simulink model "EPT"  (R2019b)
settings: Solver=FixedStepDiscrete  StartTime=0.0  StopTime=5  FixedStep=0.005  RelTol=1e-3  EnableMultiTasking=on
PreLoadFcn:
  | try, model_open; catch, disp('Error occurred while executing model pre-load callback: model_open.m'); disp('Please assure that the MATLAB working directory is set to the model directory before opening.'); end
InitFcn:
  | try, model_open; catch, end
undefined symbols (not defined in the file or in its folder): Bridge, GCM, H, ln, raptor_get_param_eval, raptor_get_safe_string, raptor_xcp_function
libraries: Raptor_lib x2810, simulink x374, hdlsllib x19
(part 20 of 45)

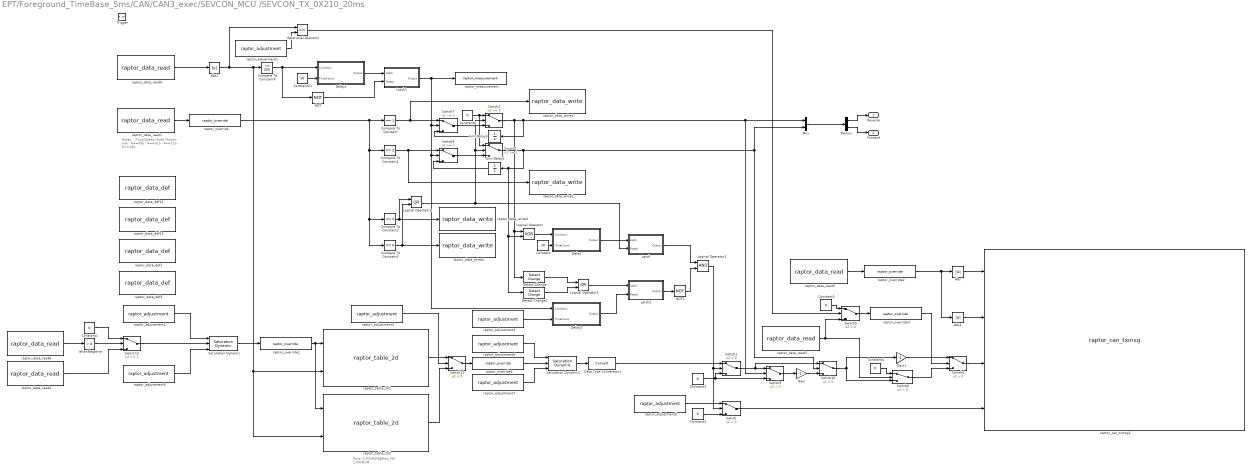
== system EPT/Foreground_TimeBase_5ms/CAN/CAN3_exec/SEVCON_MCU /SEVCON_TX_0X210_20ms  ==
  note: Note:
      | 0:FOXNUM@New_FW
      | 1:FOXNUM
  note: Notes :
      | - Torq/Speed Mode Chosen one
      | - N==00b
      | - R==01b
      | - P==11b
      | - D==10b
  Trigger : TriggerPort  VariantControl=Variant  PortDimensions=1
  Abs : Abs
  Abs1 : Abs
  Abs2 : Abs
  Compare To Constant : simulink/Logic and Bit Operations/Compare To Constant  relop===  const=1  OutDataTypeStr=boolean
  Compare To Constant1 : simulink/Logic and Bit Operations/Compare To Constant  relop===  const=2  OutDataTypeStr=boolean
  Compare To Constant2 : simulink/Logic and Bit Operations/Compare To Constant  relop===  const=3  OutDataTypeStr=boolean
  Compare To Constant3 : simulink/Logic and Bit Operations/Compare To Constant  relop===  const=0  OutDataTypeStr=boolean
  Compare To Constant4 : simulink/Logic and Bit Operations/Compare To Constant  relop=<=  const=200  OutDataTypeStr=boolean
  Constant : Constant  Value=10
  Constant{1..5} (5 alike) : Constant  Value=0
  Constant21 : Constant  Value=10
  Constant6 : Constant  Value=0  OutDataTypeStr=boolean
  Data Type Conversion1 : DataTypeConversion
  Delay : Subsystem
  Delay1 : Subsystem
  Delay3 : Subsystem
  Demux : Demux  Outputs=2
  Detect Change : simulink/Logic and Bit Operations/Detect Change  vinit=0  OutDataTypeStr=boolean
  Detect Change1 : simulink/Logic and Bit Operations/Detect Change  vinit=0  OutDataTypeStr=boolean
  Gain : Gain  Gain=-1
  Gain1 : Gain  Gain=-1
  IsNonNegative : simulink/Logic and Bit Operations/Compare To Zero  relop=>  OutDataTypeStr=boolean
  Latch : Subsystem
  Latch1 : Subsystem
  Latch2 : Subsystem
  Logical Operator : Logic  Operator=XOR  AllPortsSameDT=off  OutDataTypeStr=boolean
  Logical Operator1 : Logic  Operator=OR  AllPortsSameDT=off  OutDataTypeStr=boolean
  Logical Operator2 : Logic  Operator=OR  AllPortsSameDT=off  OutDataTypeStr=boolean
  Logical Operator3 : Logic  AllPortsSameDT=off  OutDataTypeStr=boolean
  Mux : Mux  Inputs=2
  NOT : Logic  Operator=NOT  IconShape=distinctive  AllPortsSameDT=off  OutDataTypeStr=boolean
  NOT1 : Logic  Operator=NOT  IconShape=distinctive  AllPortsSameDT=off  OutDataTypeStr=boolean
  Relational Operator : RelationalOperator  Operator=<=  OutDataTypeStr=boolean  RndMeth=Simplest
  Saturation Dynamic : simulink/Discontinuities/Saturation Dynamic  OutMin=[]  OutMax=[]  OutDataTypeStr=Inherit: Same as second input  OutDataType=fixdt(1, 16)  OutScaling=2^-10  DoSatur=off
  Saturation Dynamic1 : simulink/Discontinuities/Saturation Dynamic  OutMin=[]  OutMax=[]  OutDataTypeStr=Inherit: Same as second input  OutDataType=fixdt(1, 16)  OutScaling=2^-10  DoSatur=off
  Switch{,1,4..6,9..11} (8 alike) : Switch  Criteria=u2 > Threshold
  Switch{2..3,7..8,12} (5 alike) : Switch  Threshold=1
  Unit Delay1 : UnitDelay  SampleTime=-1  HasFrameUpgradeWarning=on
  Unit Delay3 : UnitDelay  SampleTime=-1  HasFrameUpgradeWarning=on
  raptor_adjustment1 : Raptor_lib/Data Storage/raptor_adjustment  paramName='Cal_Regen_Speed'  nameSource=Parameter  initValue=1000  dataType=double  storage=Calibration  calDispType=Number  calEnum={'False', 'True'}  calGain=1.0  calOffset=0.0  calMax=inf  calMin=-inf  calFormat='-1'  calUnit=''  calHelp=''  calAccess=1  calFunction=raptor_xcp_function(gcb)  calDispHeaders=off  calColHeaders={'Col1' 'Col2' 'Col3'}  calRowHeaders={'Row1' 'Row2' 'Row3'}
      settings: SourceProductName=Raptor
  raptor_adjustment2 : Raptor_lib/Data Storage/raptor_adjustment  paramName='Cal_TorqueMax'  nameSource=Parameter  initValue=150  dataType=double  storage=Calibration  calDispType=Number  calEnum={'False', 'True'}  calGain=1.0  calOffset=0.0  calMax=150  calMin=-150  calFormat='-1'  calUnit=''  calHelp=''  calAccess=1  calFunction=raptor_xcp_function(gcb)  calDispHeaders=off  calColHeaders={'Col1' 'Col2' 'Col3'}  calRowHeaders={'Row1' 'Row2' 'Row3'}
      settings: SourceProductName=Raptor
  raptor_adjustment3 : Raptor_lib/Data Storage/raptor_adjustment  paramName='Cal_Motor_Select'  nameSource=Parameter  initValue=1  dataType=boolean  storage=Calibration  calDispType=Number  calEnum={'False', 'True'}  calGain=1.0  calOffset=0.0  calMax=inf  calMin=-inf  calFormat='-1'  calUnit=''  calHelp=''  calAccess=1  calFunction=raptor_xcp_function(gcb)  calDispHeaders=off  calColHeaders={'Col1' 'Col2' 'Col3'}  calRowHeaders={'Row1' 'Row2' 'Row3'}
      settings: SourceProductName=Raptor
  raptor_adjustment4 : Raptor_lib/Data Storage/raptor_adjustment  paramName='Cal_Torque_Output_DelayTimes'  nameSource=Parameter  initValue=10  dataType=double  storage=Calibration  calDispType=Number  calEnum={'False', 'True'}  calGain=1.0  calOffset=0.0  calMax=inf  calMin=-inf  calFormat='-1'  calUnit=''  calHelp=''  calAccess=1  calFunction=raptor_xcp_function(gcb)  calDispHeaders=off  calColHeaders={'Col1' 'Col2' 'Col3'}  calRowHeaders={'Row1' 'Row2' 'Row3'}
      settings: SourceProductName=Raptor
  raptor_adjustment5 : Raptor_lib/Data Storage/raptor_adjustment  paramName='Cmd_Throttle_Inlet_voltage'  nameSource=Parameter  initValue=3  dataType=double  storage=Calibration  calDispType=Number  calEnum={'False', 'True'}  calGain=1.0  calOffset=0.0  calMax=inf  calMin=0  calFormat='-1'  calUnit=''  calHelp=''  calAccess=1  calFunction=raptor_xcp_function(gcb)  calDispHeaders=off  calColHeaders={'Col1' 'Col2' 'Col3'}  calRowHeaders={'Row1' 'Row2' 'Row3'}
      settings: SourceProductName=Raptor
  raptor_adjustment6 : Raptor_lib/Data Storage/raptor_adjustment  paramName='Cal_Cmd_Torque_Percentage_Max'  nameSource=Parameter  initValue=100  dataType=double  storage=Calibration  calDispType=Number  calEnum={'False', 'True'}  calGain=1.0  calOffset=0.0  calMax=inf  calMin=-inf  calFormat='-1'  calUnit=''  calHelp=''  calAccess=1  calFunction=raptor_xcp_function(gcb)  calDispHeaders=off  calColHeaders={'Col1' 'Col2' 'Col3'}  calRowHeaders={'Row1' 'Row2' 'Row3'}
      settings: SourceProductName=Raptor
  raptor_adjustment7 : Raptor_lib/Data Storage/raptor_adjustment  paramName='Cal_Cmd_Torque_Percentage_Min'  nameSource=Parameter  initValue=0  dataType=double  storage=Calibration  calDispType=Number  calEnum={'False', 'True'}  calGain=1.0  calOffset=0.0  calMax=inf  calMin=-inf  calFormat='-1'  calUnit=''  calHelp=''  calAccess=1  calFunction=raptor_xcp_function(gcb)  calDispHeaders=off  calColHeaders={'Col1' 'Col2' 'Col3'}  calRowHeaders={'Row1' 'Row2' 'Row3'}
      settings: SourceProductName=Raptor
  raptor_adjustment9 : Raptor_lib/Data Storage/raptor_adjustment  paramName='Cal_TorqueMin'  nameSource=Parameter  initValue=0.00  dataType=double  storage=Calibration  calDispType=Number  calEnum={'False', 'True'}  calGain=1.0  calOffset=0.0  calMax=150  calMin=-150  calFormat='-1'  calUnit=''  calHelp=''  calAccess=1  calFunction=raptor_xcp_function(gcb)  calDispHeaders=off  calColHeaders={'Col1' 'Col2' 'Col3'}  calRowHeaders={'Row1' 'Row2' 'Row3'}
      settings: SourceProductName=Raptor
  raptor_can_txmsg1 : Raptor_lib/CAN/raptor_can_txmsg  canDefinition=struct('dbcFile', 'SEVCON_Controller_CANopen.dbc','message', 'Cmd2','comment', '','signals', {{'Cmd_Maximum_Speed_in_Reverse','Cmd_Maximum_Speed_in_Forward','Cmd_Target_Torque','Cmd_Throttle_Inlet_voltage'}},'enabled', [ 1 1 1 1;],'canBus', '''CAN3''','messageID', [ 528;],'idMask', [ 536870911;],'payloadMask', [],'payloadValue', [],'period', [ 0;],'mailbox', '','queueSize', [ 1;],'label', [ 0;],'ver', [ 2;],'showID', [ 0;],'showRaw', [ 0;],'fill', [ 0;],'editID', [ 0;],'signalOrder', [ 2;])  canBus='CAN3'  queueSize=1  payloadMask=[]  payloadValue=[]  period=0  showID=0  label=0  idMask=hex2dec('1FFFFFFF')  fill=0  id=528  showRaw=0  signalOrder=2  signalInfo={{struct('Name', 'Cmd_Throttle_Inlet_voltage','Startbit', [ 0;],'SignalSize', [ 16;],'ByteOrder', 'LittleEndian','ValueType', 'SIGNED','Class', 'int16','Signed', [ 1;],'Factor', [ 0.0039;],'Offset', [ 0;],'Min', [ 0;],'Max', [ 0;],'Units', '','Comment', '','StartBit', [ 0;]),struct('Name', 'Cmd_Target_Torque','Startbit', [ 0;],'SignalSize', [ 16;],'ByteOrder', 'LittleEndian','ValueType', 'SIGNED','Class', 'int16','Signed', [ 1;],'Factor', [ 0.1;],'Offset', [ 0;],'Min', [ 0;],'Max', [ 0;],'Units', '','Comment', '','StartBit', [ 16;]),struct('Name', 'Cmd_Maximum_Speed_in_Reverse','Startbit', [ 0;],'SignalSize', [ 16;],'ByteOrder', 'LittleEndian','ValueType', 'SIGNED','Class', 'int16','Signed', [ 1;],'Factor', [ 1;],'Offset', [ 0;],'Min', [ 0;],'Max', [ 0;],'Units', '','Comment', '','StartBit', [ 48;]),struct('Name', 'Cmd_Maximum_Speed_in_Forward','Startbit', [ 0;],'SignalSize', [ 16;],'ByteOrder', 'LittleEndian','ValueType', 'SIGNED','Class', 'int16','Signed', [ 1;],'Factor', [ 1;],'Offset', [ 0;],'Min', [ 0;],'Max', [ 0;],'Units', '','Comment', '','StartBit', [ 32;])}}
      settings: SourceProductName=Raptor
  raptor_data_def1 : Raptor_lib/Data Storage/raptor_data_def  dataName='Position_N'  initValue=0  dataType=boolean  storage=Calibration  calVisible=on  calType=Measurement  calDispType=Number  calEnum={'False', 'True'}  calGain=1.0  calOffset=0  calMin=-inf  calMax=inf  calFormat='-1'  calUnit=''  calHelp=''  calAccess=1  calFunction=raptor_xcp_function(gcb)  calDispHeaders=off  calColHeaders={'Col1' 'Col2' 'Col3'}  calRowHeaders={'Row1' 'Row2' 'Row3'}
      settings: SourceProductName=Raptor
  raptor_data_def13 : Raptor_lib/Data Storage/raptor_data_def  dataName='Position_R'  initValue=0  dataType=boolean  storage=Calibration  calVisible=on  calType=Measurement  calDispType=Number  calEnum={'False', 'True'}  calGain=1.0  calOffset=0  calMin=-inf  calMax=inf  calFormat='-1'  calUnit=''  calHelp=''  calAccess=1  calFunction=raptor_xcp_function(gcb)  calDispHeaders=off  calColHeaders={'Col1' 'Col2' 'Col3'}  calRowHeaders={'Row1' 'Row2' 'Row3'}
      settings: SourceProductName=Raptor
  raptor_data_def14 : Raptor_lib/Data Storage/raptor_data_def  dataName='Position_D'  initValue=0  dataType=boolean  storage=Calibration  calVisible=on  calType=Measurement  calDispType=Number  calEnum={'False', 'True'}  calGain=1.0  calOffset=0  calMin=-inf  calMax=inf  calFormat='-1'  calUnit=''  calHelp=''  calAccess=1  calFunction=raptor_xcp_function(gcb)  calDispHeaders=off  calColHeaders={'Col1' 'Col2' 'Col3'}  calRowHeaders={'Row1' 'Row2' 'Row3'}
      settings: SourceProductName=Raptor
  raptor_data_def3 : Raptor_lib/Data Storage/raptor_data_def  dataName='Position_P'  initValue=0  dataType=boolean  storage=Calibration  calVisible=on  calType=Measurement  calDispType=Number  calEnum={'False', 'True'}  calGain=1.0  calOffset=0  calMin=-inf  calMax=inf  calFormat='-1'  calUnit=''  calHelp=''  calAccess=1  calFunction=raptor_xcp_function(gcb)  calDispHeaders=off  calColHeaders={'Col1' 'Col2' 'Col3'}  calRowHeaders={'Row1' 'Row2' 'Row3'}
      settings: SourceProductName=Raptor
  raptor_data_read1 : Raptor_lib/Data Storage/raptor_data_read  dataName='ECHS_GEAR_CMD'  dataShape=Scalar  idxSource=Input  idxRow=1  idxCol=1
      settings: SourceProductName=Raptor
  raptor_data_read2 : Raptor_lib/Data Storage/raptor_data_read  dataName='ECHS_TRQ_CMD'  dataShape=Scalar  idxSource=Input  idxRow=1  idxCol=1
      settings: SourceProductName=Raptor
  raptor_data_read3 : Raptor_lib/Data Storage/raptor_data_read  dataName='ECHS_REG_MODE_REQ'  dataShape=Scalar  idxSource=Input  idxRow=1  idxCol=1
      settings: SourceProductName=Raptor
  raptor_data_read4 : Raptor_lib/Data Storage/raptor_data_read  dataName='Read_Motor_Speed'  dataShape=Scalar  idxSource=Input  idxRow=1  idxCol=1
      settings: SourceProductName=Raptor
  raptor_data_read5 : Raptor_lib/Data Storage/raptor_data_read  dataName='ECHS_SPD_CMD'  dataShape=Scalar  idxSource=Input  idxRow=1  idxCol=1
      settings: SourceProductName=Raptor
  raptor_data_read6 : Raptor_lib/Data Storage/raptor_data_read  dataName='HV_Off_State'  dataShape=Scalar  idxSource=Input  idxRow=1  idxCol=1
      settings: SourceProductName=Raptor
  raptor_data_write1 : Raptor_lib/Data Storage/raptor_data_write  dataName='Position_D'  dataShape=Scalar  idxSource=Input Port  idxRow=1  idxCol=1
      settings: SourceProductName=Raptor
  raptor_data_write2 : Raptor_lib/Data Storage/raptor_data_write  dataName='Position_R'  dataShape=Scalar  idxSource=Input Port  idxRow=1  idxCol=1
      settings: SourceProductName=Raptor
  raptor_data_write3 : Raptor_lib/Data Storage/raptor_data_write  dataName='Position_P'  dataShape=Scalar  idxSource=Input Port  idxRow=1  idxCol=1
      settings: SourceProductName=Raptor
  raptor_data_write4 : Raptor_lib/Data Storage/raptor_data_write  dataName='Position_N'  dataShape=Scalar  idxSource=Input Port  idxRow=1  idxCol=1
      settings: SourceProductName=Raptor
  raptor_measurement : Raptor_lib/Data Storage/raptor_measurement  paramName='FlagSpeedLow'  nameSource=Parameter  calDispType=Number  calEnum={'False', 'True'}  calGain=1.0  calOffset=0.0  calMax=inf  calMin=-inf  calFormat='-1'  calUnit=''  calHelp=''  calAccess=1  calFunction=raptor_xcp_function(gcb)  calVisible=on
      settings: SourceProductName=Raptor
  raptor_override : Raptor_lib/Data Storage/raptor_override  paramName='Cal_Cmd_F_R_Switch'  nameSource=Parameter  measurement=None  calDispType=Number  calEnum={'False', 'True'}  calGain=1.0  calOffset=0.0  calMax=inf  calMin=-inf  calFormat='-1'  calUnit=''  calHelp=''  calAccess=1  calFunction=[raptor_xcp_function(gcb) '|' raptor_get_param_eval(gcb, 'paramName') '_Override']
      settings: SourceProductName=Raptor
  raptor_override1 : Raptor_lib/Data Storage/raptor_override  paramName='Cal_Cmd_Target_Torque'  nameSource=Parameter  measurement=None  calDispType=Number  calEnum={'False', 'True'}  calGain=1.0  calOffset=0.0  calMax=inf  calMin=-inf  calFormat='-1'  calUnit=''  calHelp=''  calAccess=1  calFunction=[raptor_xcp_function(gcb) '|' raptor_get_param_eval(gcb, 'paramName') '_Override']
      settings: SourceProductName=Raptor
  raptor_override2 : Raptor_lib/Data Storage/raptor_override  paramName='Cal_Cmd_SpeedLimit'  nameSource=Parameter  measurement=None  calDispType=Number  calEnum={'False', 'True'}  calGain=1.0  calOffset=0.0  calMax=inf  calMin=-inf  calFormat='-1'  calUnit=''  calHelp=''  calAccess=1  calFunction=[raptor_xcp_function(gcb) '|' raptor_get_param_eval(gcb, 'paramName') '_Override']
      settings: SourceProductName=Raptor
  raptor_override3 : Raptor_lib/Data Storage/raptor_override  paramName='Cal_Cmd_Regen'  nameSource=Parameter  measurement=None  calDispType=Number  calEnum={'False', 'True'}  calGain=1.0  calOffset=0.0  calMax=inf  calMin=-inf  calFormat='-1'  calUnit=''  calHelp=''  calAccess=1  calFunction=[raptor_xcp_function(gcb) '|' raptor_get_param_eval(gcb, 'paramName') '_Override']
      settings: SourceProductName=Raptor
  raptor_override4 : Raptor_lib/Data Storage/raptor_override  paramName='Cal_Cmd_Torque_Percentage'  nameSource=Parameter  measurement=None  calDispType=Number  calEnum={'False', 'True'}  calGain=1.0  calOffset=0.0  calMax=inf  calMin=-inf  calFormat='-1'  calUnit=''  calHelp=''  calAccess=1  calFunction=[raptor_xcp_function(gcb) '|' raptor_get_param_eval(gcb, 'paramName') '_Override']
      settings: SourceProductName=Raptor
  raptor_table_2d1 : Raptor_lib/Table Lookup/raptor_table_2d  dataName='FOXNUM'  initValue=|  dataType=double  storage=Calibration  initValueX="[0\t500\t1000\t1500\t2000\t2500\t3000\t3500\t4000\t4500\t5000\t6000]"  initValueY="[0\t5\t10\t20\t30\t40\t50\t60\t70\t80\t90\t100\t110\t120\t130]"  dataTypeXY=double  storageXY=Calibration  calVisible=on  showTable=off  calGain=1.0  calOffset=0.0  calMax=Inf  calMin=-Inf  calFormat='-1'  calUnit=''  calHelp=''  showBreakpointX=off  dataNameX=[]  calGainX=1.0  calOffsetX=0.0  calMaxX=Inf  calMinX=-Inf  calFormatX='-1'  calUnitX=''  calHelpX=''  showBreakpointY=off  dataNameY=[]  calGainY=1.0  calOffsetY=0.0  calMaxY=Inf  calMinY=-Inf  calFormatY='-1'  calUnitY=''  calHelpY=''  calAccess=1  calFunction=raptor_xcp_function(gcb)  measureEnable=off  mName=[raptor_get_param_eval(gcb,'dataName'), '_Output']
      | [0	0	0	0	0	0	0	0	0	0	0	0
      | 26	26	26	23	21	17.5000000000000	21	19.1000000000000	17.7000000000000	17.3000000000000	16	16
      | 34	34	35	33.1000000000000	30	30	28.3000000000000	26.4000000000000	26	25	24	24
      | 44.4000000000000	44.4000000000000	46	43	39	38.3000000000000	37	35.3000000000000	34	32.5000000000000	38.5000000000000	38.5000000000000
      | 51.2000000000000	51.2000000000000	53.7000000000000	50	46	44.5000000000000	42.7000000000000	41.1000000000000	46.5000000000000	54.5000000000000	70	70
      | 59	59	60.4000000000000	56	51	50.2000000000000	48	53.9000000000000	70	100	100	100
      | 64.8000000000000	64.8000000000000	66	61	55	55	54.6000000000000	80	100	100	100	100
      | 70.3000000000000	70.3000000000000	71	65.5000000000000	58.9000000000000	59	75	100	100	100	100	100
      | 75.3000000000000	75.3000000000000	75.4000000000000	70	62.6000000000000	64.5000000000000	100	100	100	100	100	100
      | 80	80	79.9000000000000	74	68.6000000000000	85	100	100	100	100	100	100
      | 84.8000000000000	84.8000000000000	84.2000000000000	78	71.7000000000000	100	100	100	100	100	100	100
      | 89.1000000000000	89.1000000000000	88.4000000000000	81.5000000000000	81.2000000000000	100	100	100	100	100	100	100
      | 96.1000000000000	96.1000000000000	95	84	100	100	100	100	100	100	100	100
      | 100	100	100	90	100	100	100	100	100	100	100	100
      | 100	100	100	100	100	100	100	100	100	100	100	100]
      settings: SourceProductName=Raptor
  raptor_table_2d2 : Raptor_lib/Table Lookup/raptor_table_2d  dataName='AC_35'  initValue=|  dataType=double  storage=Calibration  initValueX="[0\t500\t1000\t1500\t2000\t2500\t3000\t3500\t4000\t4500\t5000\t5500\t6000\t6500]"  initValueY=|  dataTypeXY=double  storageXY=Calibration  calVisible=on  showTable=off  calGain=1.0  calOffset=0.0  calMax=Inf  calMin=-Inf  calFormat='-1'  calUnit=''  calHelp=''  showBreakpointX=off  dataNameX=[]  calGainX=1.0  calOffsetX=0.0  calMaxX=Inf  calMinX=-Inf  calFormatX='-1'  calUnitX=''  calHelpX=''  showBreakpointY=off  dataNameY=[]  calGainY=1.0  calOffsetY=0.0  calMaxY=Inf  calMinY=-Inf  calFormatY='-1'  calUnitY=''  calHelpY=''  calAccess=1  calFunction=raptor_xcp_function(gcb)  measureEnable=off  mName=[raptor_get_param_eval(gcb,'dataName'), '_Output']
      initValue=|
      | [0	0	0	0	0	0	0	0	0	0	0	0	0	0
      | 4.8 	4.8 	4.9 	4.9 	5.1 	5.0 	5.0 	5.1 	5.0 	5.0 	5.1 	5.1 	5.1 	5.1 
      | 8.3 	8.3 	8.9 	8.7 	9.5 	8.5 	8.8 	8.7 	8.7 	8.7 	8.7 	8.7 	8.7 	8.7 
      | 11.7 	11.7 	12.2 	12.1 	13.5 	11.8 	12.7 	12.0 	12.0 	12.4 	12.7 	13.0 	13.2 	13.2 
      | 15.0 	15.0 	15.5 	15.5 	17.5 	15.0 	16.5 	15.3 	15.3 	16.1 	16.7 	17.3 	17.6 	17.6 
      | 18.7 	18.7 	19.3 	19.3 	21.8 	18.5 	20.4 	19.1 	19.8 	20.7 	21.4 	23.6 	20.3 	20.3 
      | 22.3 	22.3 	23.0 	23.0 	26.0 	22.0 	24.3 	22.9 	24.3 	25.2 	26.0 	23.6 	20.3 	20.3 
      | 25.9 	25.9 	26.7 	26.4 	29.8 	25.5 	27.8 	27.0 	29.1 	30.6 	28.0 	23.6 	20.3 	20.3 
      | 29.5 	29.5 	30.4 	29.8 	33.5 	29.0 	31.3 	31.0 	33.9 	35.0 	28.0 	23.6 	20.3 	20.3 
      | 32.7 	32.7 	33.5 	33.0 	36.8 	32.0 	34.7 	35.5 	39.5 	35.0 	28.0 	23.6 	20.3 	20.3 
      | 35.9 	35.9 	36.5 	36.1 	40.0 	35.0 	38.0 	40.0 	45.0 	35.0 	28.0 	23.6 	20.3 	20.3 
      | 39.5 	39.5 	40.1 	39.6 	43.8 	38.5 	41.5 	45.0 	45.0 	35.0 	28.0 	23.6 	20.3 	20.3 
      | 43.0 	43.0 	43.6 	43.1 	47.5 	42.0 	45.0 	50.0 	45.0 	35.0 	28.0 	23.6 	20.3 	20.3 
      | 46.7 	46.7 	47.2 	46.9 	50.8 	46.0 	49.5 	55.0 	45.0 	35.0 	28.0 	23.6 	20.3 	20.3 
      | 50.4 	50.4 	50.8 	50.6 	54.0 	50.0 	54.0 	55.0 	45.0 	35.0 	28.0 	23.6 	20.3 	20.3 
      | 53.2 	53.2 	53.5 	53.1 	56.5 	53.5 	59.0 	55.0 	45.0 	35.0 	28.0 	23.6 	20.3 	20.3 
      | 56.0 	56.0 	56.1 	55.6 	59.0 	57.0 	64.0 	55.0 	45.0 	35.0 	28.0 	23.6 	20.3 	20.3 
      | 58.4 	58.4 	58.5 	58.2 	61.3 	59.5 	70.0 	55.0 	45.0 	35.0 	28.0 	23.6 	20.3 	20.3 
      | 60.8 	60.8 	60.9 	60.7 	63.5 	62.0 	70.0 	55.0 	45.0 	35.0 	28.0 	23.6 	20.3 	20.3 
      | 63.0 	63.0 	63.0 	62.9 	65.4 	66.0 	70.0 	55.0 	45.0 	35.0 	28.0 	23.6 	20.3 	20.3 
      | 65.2 	65.2 	65.1 	65.0 	67.3 	70.0 	70.0 	55.0 	45.0 	35.0 	28.0 	23.6 	20.3 	20.3 
      | 67.6 	67.6 	67.6 	67.5 	69.2 	74.5 	70.0 	55.0 	45.0 	35.0 	28.0 	23.6 	20.3 	20.3 
      | 70.0 	70.0 	70.0 	70.0 	71.0 	79.0 	70.0 	55.0 	45.0 	35.0 	28.0 	23.6 	20.3 	20.3 
      | 71.3 	71.3 	71.4 	71.3 	72.4 	79.0 	70.0 	55.0 	45.0 	35.0 	28.0 	23.6 	20.3 	20.3 
      | 72.6 	72.6 	72.7 	72.6 	73.8 	79.0 	70.0 	55.0 	45.0 	35.0 	28.0 	23.6 	20.3 	20.3 
      | 74.1 	74.1 	74.1 	74.0 	75.1 	79.0 	70.0 	55.0 	45.0 	35.0 	28.0 	23.6 	20.3 	20.3 
      | 75.5 	75.5 	75.4 	75.4 	76.4 	79.0 	70.0 	55.0 	45.0 	35.0 	28.0 	23.6 	20.3 	20.3 
      | 76.8 	76.8 	76.7 	76.7 	77.7 	79.0 	70.0 	55.0 	45.0 	35.0 	28.0 	23.6 	20.3 	20.3 
      | 78.0 	78.0 	78.0 	78.0 	79.0 	79.0 	70.0 	55.0 	45.0 	35.0 	28.0 	23.6 	20.3 	20.3 
      | 80.4 	80.4 	80.7 	80.7 	81.0 	79.0 	70.0 	55.0 	45.0 	35.0 	28.0 	23.6 	20.3 	20.3 
      | 83.8 	83.8 	84.0 	84.0 	81.0 	79.0 	70.0 	55.0 	45.0 	35.0 	28.0 	23.6 	20.3 	20.3 
      | ]
      initValueY=|
      | [0	5	10	15	20	25	30	35	40	45	50	55	60	65	70	75	80	85	90	95	100	105	110	115	120	125	130	135	140	150	160
      | ]
      settings: SourceProductName=Raptor
  Reverse : Outport  VectorParamsAs1DForOutWhenUnconnected=off
  Forward : Outport  Port=2  VectorParamsAs1DForOutWhenUnconnected=off
  wires:
  Latch1/1(Output) -> Delay3/1(Condition), Switch8/2, Switch7/2, raptor_measurement/1
  raptor_adjustment9/1 -> Saturation Dynamic/3
  raptor_override1/1 -> raptor_table_2d2/1, raptor_table_2d1/1
  Gain/1 -> Switch10/3
  raptor_adjustment2/1 -> Saturation Dynamic/1
  Latch/1(Output) -> Logical Operator3/1
  Abs2/1 -> Relational Operator/1, raptor_table_2d2/2, raptor_table_2d1/2, Compare To Constant4/1
  Switch9/1 -> Gain/1
  Latch2/1(Output) -> NOT1/1
  raptor_data_read4/1 -> Abs2/1
  Logical Operator1/1 -> Latch2/1(Latch)
  Detect Change1/1 -> Logical Operator1/2
  Constant21/1 -> Delay1/2(TimeCount)
  NOT1/1 -> Logical Operator3/2
  Switch8/1 -> Switch3/3
  Logical Operator2/1 -> Latch/2(Reset), Switch3/2, Switch2/2
  Switch3/1 -> Unit Delay1/1, Detect Change1/1, Logical Operator/2, Switch10/2, Mux/2
  Data Type Conversion1/1 -> Switch1/1
  Detect Change/1 -> Logical Operator1/1
  Switch1/1 -> Switch10/1, Switch9/1
  Logical Operator3/1 -> Switch1/2, Switch/2
  raptor_data_read1/1 -> raptor_override/1
  Switch2/1 -> Detect Change/1, Logical Operator/1, Unit Delay3/1, Switch9/2, Mux/1
  Switch7/1 -> Switch2/3
  Logical Operator/1 -> Delay/1(Condition)
  NOT/1 -> Latch1/2(Reset)
  Compare To Constant4/1 -> Delay1/1(Condition), NOT/1
  Unit Delay1/1 -> Switch8/3
  Delay1/1(Output) -> Latch1/1(Latch)
  Compare To Constant/1 -> raptor_data_write2/1, Switch7/1
  Compare To Constant1/1 -> raptor_data_write1/1, Switch8/1
  Saturation Dynamic/1 -> raptor_override1/1
  Switch/1 -> raptor_can_txmsg1/4
  Unit Delay3/1 -> Switch7/3
  Compare To Constant3/1 -> Logical Operator2/2, raptor_data_write4/1
  Abs1/1 -> raptor_can_txmsg1/2
  raptor_adjustment5/1 -> Switch/1
  raptor_override2/1 -> Abs1/1, Abs/1
  Compare To Constant2/1 -> Logical Operator2/1, raptor_data_write3/1
  Constant/1 -> Delay/2(TimeCount)
  raptor_override/1 -> Compare To Constant3/1, Compare To Constant2/1, Compare To Constant1/1, Compare To Constant/1
  raptor_data_read5/1 -> raptor_override2/1
  Delay/1(Output) -> Latch/1(Latch)
  Abs/1 -> raptor_can_txmsg1/1
  Switch10/1 -> Switch6/3, Gain1/1
  Switch4/1 -> raptor_can_txmsg1/3
  Gain1/1 -> Switch4/1
  Demux/1 -> Reverse/1
  Demux/2 -> Forward/1
  Mux/1 -> Demux/1
  Delay3/1(Output) -> Latch2/2(Reset)
  raptor_adjustment4/1 -> Delay3/2(TimeCount)
  raptor_data_read3/1 -> Switch5/3, Switch6/2
  Switch5/1 -> raptor_override3/1
  Switch6/1 -> Switch4/3
  raptor_override3/1 -> Switch4/2
  raptor_adjustment1/1 -> Relational Operator/2
  Relational Operator/1 -> Switch5/2
  Switch11/1 -> raptor_override4/1
  raptor_table_2d1/1 -> Switch11/1
  raptor_table_2d2/1 -> Switch11/3
  raptor_adjustment3/1 -> Switch11/2
  raptor_override4/1 -> Saturation Dynamic1/2
  Saturation Dynamic1/1 -> Data Type Conversion1/1
  raptor_adjustment6/1 -> Saturation Dynamic1/1
  raptor_adjustment7/1 -> Saturation Dynamic1/3
  raptor_data_read2/1 -> Switch12/3
  Switch12/1 -> Saturation Dynamic/2
  raptor_data_read6/1 -> IsNonNegative/1
  IsNonNegative/1 -> Switch12/2
  Constant1/1 -> Switch12/1
  Constant2/1 -> Switch/3
  Constant3/1 -> Switch9/3, Switch1/3
  Constant4/1 -> Switch6/1
  Constant5/1 -> Switch5/1
  Constant6/1 -> Switch2/1, Switch3/1

== system EPT/Foreground_TimeBase_5ms/CAN/CAN3_exec/SEVCON_MCU /SEVCON_TX_0X211_20ms  ==
  Cmd_Reverse_Switch : Inport
  Cmd_Forward_Switch : Inport  Port=2
  Trigger : TriggerPort  VariantControl=Variant  PortDimensions=1
  raptor_adjustment1 : Raptor_lib/Data Storage/raptor_adjustment  paramName='Cmd_Handbrake_Switch'  nameSource=Parameter  initValue=0.00  dataType=boolean  storage=Calibration  calDispType=Number  calEnum={'False', 'True'}  calGain=1.0  calOffset=0.0  calMax=inf  calMin=-inf  calFormat='-1'  calUnit=''  calHelp=''  calAccess=1  calFunction=raptor_xcp_function(gcb)  calDispHeaders=off  calColHeaders={'Col1' 'Col2' 'Col3'}  calRowHeaders={'Row1' 'Row2' 'Row3'}
      settings: SourceProductName=Raptor
  raptor_adjustment3 : Raptor_lib/Data Storage/raptor_adjustment  paramName='Cmd_Seat_Switch'  nameSource=Parameter  initValue=1  dataType=boolean  storage=Calibration  calDispType=Number  calEnum={'False', 'True'}  calGain=1.0  calOffset=0.0  calMax=inf  calMin=-inf  calFormat='-1'  calUnit=''  calHelp=''  calAccess=1  calFunction=raptor_xcp_function(gcb)  calDispHeaders=off  calColHeaders={'Col1' 'Col2' 'Col3'}  calRowHeaders={'Row1' 'Row2' 'Row3'}
      settings: SourceProductName=Raptor
  raptor_can_txmsg : Raptor_lib/CAN/raptor_can_txmsg  canDefinition=struct('dbcFile', 'SEVCON_Controller_CANopen.dbc','message', 'Cmd1','comment', '','signals', {{'Cmd_Handbrake_Switch','Cmd_Seat_Switch','Cmd_Reverse_Switch','Cmd_Forward_Switch','Cmd_Battery_Dischg_Current_Limit','Cmd_Battery_Chg_Current_Limit'}},'enabled', [ 1 1 1 1 1 1;],'canBus', '''CAN3''','messageID', [ 529;],'idMask', [ 536870911;],'payloadMask', [],'payloadValue', [],'period', [ 0;],'mailbox', '','queueSize', [ 1;],'label', [ 0;],'ver', [ 2;],'showID', [ 0;],'showRaw', [ 0;],'fill', [ 0;],'editID', [ 0;],'signalOrder', [ 2;])  canBus='CAN3'  queueSize=1  payloadMask=[]  payloadValue=[]  period=0  showID=0  label=0  idMask=hex2dec('1FFFFFFF')  fill=0  id=529  showRaw=0  signalOrder=2  signalInfo={{struct('Name', 'Cmd_Seat_Switch','Startbit', [ 0;],'SignalSize', [ 1;],'ByteOrder', 'LittleEndian','ValueType', 'UNSIGNED','Class', 'uint8','Signed', [ 0;],'Factor', [ 1;],'Offset', [ 0;],'Min', [ 0;],'Max', [ 0;],'Units', '','Comment', '','StartBit', [ 34;]),struct('Name', 'Cmd_Reverse_Switch','Startbit', [ 0;],'SignalSize', [ 1;],'ByteOrder', 'LittleEndian','ValueType', 'UNSIGNED','Class', 'uint8','Signed', [ 0;],'Factor', [ 1;],'Offset', [ 0;],'Min', [ 0;],'Max', [ 0;],'Units', '','Comment', '','StartBit', [ 33;]),struct('Name', 'Cmd_Handbrake_Switch','Startbit', [ 0;],'SignalSize', [ 1;],'ByteOrder', 'LittleEndian','ValueType', 'UNSIGNED','Class', 'uint8','Signed', [ 0;],'Factor', [ 1;],'Offset', [ 0;],'Min', [ 0;],'Max', [ 0;],'Units', '','Comment', '','StartBit', [ 35;]),struct('Name', 'Cmd_Forward_Switch','Startbit', [ 0;],'SignalSize', [ 1;],'ByteOrder', 'LittleEndian','ValueType', 'UNSIGNED','Class', 'uint8','Signed', [ 0;],'Factor', [ 1;],'Offset', [ 0;],'Min', [ 0;],'Max', [ 0;],'Units', '','Comment', '','StartBit', [ 32;]),struct('Name', 'Cmd_Battery_Dischg_Current_Limit','Startbit', [ 0;],'SignalSize', [ 16;],'ByteOrder', 'LittleEndian','ValueType', 'SIGNED','Class', 'int16','Signed', [ 1;],'Factor', [ 1;],'Offset', [ 0;],'Min', [ 0;],'Max', [ 0;],'Units', '','Comment', '','StartBit', [ 16;]),struct('Name', 'Cmd_Battery_Chg_Current_Limit','Startbit', [ 0;],'SignalSize', [ 16;],'ByteOrder', 'LittleEndian','ValueType', 'SIGNED','Class', 'int16','Signed', [ 1;],'Factor', [ 1;],'Offset', [ 0;],'Min', [ 0;],'Max', [ 0;],'Units', '','Comment', '','StartBit', [ 0;])}}
      settings: SourceProductName=Raptor
  raptor_data_def11 : Raptor_lib/Data Storage/raptor_data_def  dataName='Cmd_Battery_Chg_Current_Limit'  initValue=450  dataType=double  storage=Volatile (RAM)  calVisible=on  calType=Measurement  calDispType=Number  calEnum={'False', 'True'}  calGain=1.0  calOffset=0  calMin=-inf  calMax=inf  calFormat='-1'  calUnit=''  calHelp=''  calAccess=1  calFunction=raptor_xcp_function(gcb)  calDispHeaders=off  calColHeaders={'Col1' 'Col2' 'Col3'}  calRowHeaders={'Row1' 'Row2' 'Row3'}
      settings: SourceProductName=Raptor
  raptor_data_def30 : Raptor_lib/Data Storage/raptor_data_def  dataName='Cmd_Battery_Dischg_Current_Limit'  initValue=-450  dataType=double  storage=Volatile (RAM)  calVisible=on  calType=Measurement  calDispType=Number  calEnum={'False', 'True'}  calGain=1.0  calOffset=0  calMin=-inf  calMax=inf  calFormat='-1'  calUnit=''  calHelp=''  calAccess=1  calFunction=raptor_xcp_function(gcb)  calDispHeaders=off  calColHeaders={'Col1' 'Col2' 'Col3'}  calRowHeaders={'Row1' 'Row2' 'Row3'}
      settings: SourceProductName=Raptor
  raptor_data_read3 : Raptor_lib/Data Storage/raptor_data_read  dataName='Cmd_Battery_Dischg_Current_Limit'  dataShape=Scalar  idxSource=Input  idxRow=1  idxCol=1
      settings: SourceProductName=Raptor
  raptor_data_read4 : Raptor_lib/Data Storage/raptor_data_read  dataName='Cmd_Battery_Chg_Current_Limit'  dataShape=Scalar  idxSource=Input  idxRow=1  idxCol=1
      settings: SourceProductName=Raptor
  wires:
  raptor_data_read3/1 -> raptor_can_txmsg/5
  raptor_adjustment3/1 -> raptor_can_txmsg/2
  raptor_adjustment1/1 -> raptor_can_txmsg/1
  raptor_data_read4/1 -> raptor_can_txmsg/6
  Cmd_Reverse_Switch/1 -> raptor_can_txmsg/3
  Cmd_Forward_Switch/1 -> raptor_can_txmsg/4

== system EPT/Foreground_TimeBase_5ms/CAN/CAN3_exec/SWCU/CountTrigger ==
  Counter : Inport
  Constant1 : Constant  Value=0
  Constant3 : Constant
  CycleTrigger : Subsystem
  Switch : Switch  Threshold=1
  Unit Delay1 : UnitDelay  SampleTime=-1  HasFrameUpgradeWarning=on
  Unit Delay2 : UnitDelay  SampleTime=-1  HasFrameUpgradeWarning=on
  Tirgger : Outport  VectorParamsAs1DForOutWhenUnconnected=off
  wires:
  Unit Delay2/1 -> Tirgger/1
  Unit Delay1/1 -> CycleTrigger/1(In1)
  CycleTrigger/1(Trigger) -> Unit Delay2/1, Switch/2
  Counter/1 -> CycleTrigger/2(In2)
  Constant1/1 -> Switch/1
  Constant3/1 -> Switch/3
  Switch/1 -> Unit Delay1/1

== system EPT/Foreground_TimeBase_5ms/CAN/CAN3_exec/SWCU/CountTrigger1 ==
  Counter : Inport
  Constant1 : Constant  Value=0
  Constant3 : Constant
  CycleTrigger : Subsystem
  Switch : Switch  Threshold=1
  Unit Delay1 : UnitDelay  SampleTime=-1  HasFrameUpgradeWarning=on
  Unit Delay2 : UnitDelay  SampleTime=-1  HasFrameUpgradeWarning=on
  Tirgger : Outport  VectorParamsAs1DForOutWhenUnconnected=off
  wires:
  Switch/1 -> Unit Delay1/1
  Constant3/1 -> Switch/3
  Constant1/1 -> Switch/1
  Counter/1 -> CycleTrigger/2(In2)
  CycleTrigger/1(Trigger) -> Switch/2, Unit Delay2/1
  Unit Delay1/1 -> CycleTrigger/1(In1)
  Unit Delay2/1 -> Tirgger/1

== system EPT/Foreground_TimeBase_5ms/CAN/CAN3_exec/SWCU/EPT to SWCU Enable Control ==
  note: 0:Normal(Power Output)
      | 1: Power Standby Mode
  note: 0: HV OFF
      | 1: HV Enable
  note: 0: Unused;
      | 1: Power Steady Mode;
      | 2: Power Dynamic Mode
  Trigger : TriggerPort  TriggerType=falling  VariantControl=Variant  PortDimensions=1
  Compare To Constant : simulink/Logic and Bit Operations/Compare To Constant  relop===  const=3  OutDataTypeStr=boolean
  Compare To Constant1 : simulink/Logic and Bit Operations/Compare To Constant  relop===  const=1  OutDataTypeStr=boolean
  Constant7 : Constant  Value=15
  Delay : Subsystem
  EPT_SWCU_POUT_CMD : Subsystem
  Latch : Subsystem
  Logical Operator : Logic  Inputs=3  AllPortsSameDT=off  OutDataTypeStr=boolean
  Logical Operator2 : Logic  Operator=OR  AllPortsSameDT=off  OutDataTypeStr=boolean
  Logical Operator3 : Logic  Operator=NOR  AllPortsSameDT=off  OutDataTypeStr=boolean
  Logical Operator4 : Logic  AllPortsSameDT=off  OutDataTypeStr=boolean
  NOT : Logic  Operator=NOT  IconShape=distinctive  AllPortsSameDT=off  OutDataTypeStr=boolean
  RollingCount1 : Subsystem
  raptor_adjustment : Raptor_lib/Data Storage/raptor_adjustment  paramName='Cal_EPT_SWCU_HV_ENA_DelayTime'  nameSource=Parameter  initValue=200  dataType=double  storage=Calibration  calDispType=Number  calEnum={'False', 'True'}  calGain=1.0  calOffset=0.0  calMax=inf  calMin=-inf  calFormat='-1'  calUnit=''  calHelp=''  calAccess=1  calFunction=raptor_xcp_function(gcb)  calDispHeaders=off  calColHeaders={'Col1' 'Col2' 'Col3'}  calRowHeaders={'Row1' 'Row2' 'Row3'}
      settings: SourceProductName=Raptor
  raptor_can_txmsg : Raptor_lib/CAN/raptor_can_txmsg  canDefinition=struct('dbcFile', 'EPTvsSWCU.dbc','message', 'EPT_to_SWCU_Enable_Control','comment', '','signals', {{'EPT_READY','EPT_EW_STA','EPT_SWCU_PWR_STANDBY','EPT_SWCU_HV_ENA','EPT_HV_PROTECTED','EPT_SWCU_OUTPUT_MODE','EPT_SWCU_POUT_CMD','EPT_BPSWU_SWAP_LVL','EPT_SWCU_CTRL_CHKSUM','EPT_SWCU_CTRL_RC','EPT_SWCU_CTRL_HOST_ID'}},'enabled', [ 1 1 1 1 1 1 1 1 1 1 1;],'canBus', '''CAN3''','messageID', [ 402679028;],'idMask', [ 536870911;],'payloadMask', [],'payloadValue', [],'period', [ 0;],'mailbox', '','queueSize', [ 1;],'label', [ 0;],'ver', [ 2;],'showID', [ 0;],'showRaw', [ 0;],'fill', [ 0;],'editID', [ 0;],'signalOrder', [ 2;])  canBus='CAN3'  queueSize=1  payloadMask=[]  payloadValue=[]  period=0  showID=0  label=0  idMask=hex2dec('1FFFFFFF')  fill=0  id=402679028  showRaw=0  signalOrder=2  signalInfo={{struct('Name', 'EPT_SWCU_HV_ENA','Startbit', [ 0;],'SignalSize', [ 1;],'ByteOrder', 'LittleEndian','ValueType', 'UNSIGNED','Class', 'uint8','Signed', [ 0;],'Factor', [ 1;],'Offset', [ 0;],'Min', [ 0;],'Max', [ 0;],'Units', '','Comment', '','StartBit', [ 9;]),struct('Name', 'EPT_READY','Startbit', [ 0;],'SignalSize', [ 1;],'ByteOrder', 'LittleEndian','ValueType', 'UNSIGNED','Class', 'uint8','Signed', [ 0;],'Factor', [ 1;],'Offset', [ 0;],'Min', [ 0;],'Max', [ 0;],'Units', '','Comment', '','StartBit', [ 0;]),struct('Name', 'EPT_HV_PROTECTED','Startbit', [ 0;],'SignalSize', [ 1;],'ByteOrder', 'LittleEndian','ValueType', 'UNSIGNED','Class', 'uint8','Signed', [ 0;],'Factor', [ 1;],'Offset', [ 0;],'Min', [ 0;],'Max', [ 0;],'Units', '','Comment', '','StartBit', [ 15;]),struct('Name', 'EPT_EW_STA','Startbit', [ 0;],'SignalSize', [ 1;],'ByteOrder', 'LittleEndian','ValueType', 'UNSIGNED','Class', 'uint8','Signed', [ 0;],'Factor', [ 1;],'Offset', [ 0;],'Min', [ 0;],'Max', [ 0;],'Units', '','Comment', '','StartBit', [ 7;]),struct('Name', 'EPT_BPSWU_SWAP_LVL','Startbit', [ 0;],'SignalSize', [ 8;],'ByteOrder', 'LittleEndian','ValueType', 'UNSIGNED','Class', 'uint8','Signed', [ 0;],'Factor', [ 0.5;],'Offset', [ 0;],'Min', [ 0;],'Max', [ 0;],'Units', '%','Comment', '','StartBit', [ 40;]),struct('Name', 'EPT_SWCU_POUT_CMD','Startbit', [ 0;],'SignalSize', [ 16;],'ByteOrder', 'LittleEndian','ValueType', 'UNSIGNED','Class', 'uint16','Signed', [ 0;],'Factor', [ 0.001;],'Offset', [ 0;],'Min', [ 0;],'Max', [ 0;],'Units', 'kw','Comment', '','StartBit', [ 24;]),struct('Name', 'EPT_SWCU_OUTPUT_MODE','Startbit', [ 0;],'SignalSize', [ 2;],'ByteOrder', 'LittleEndian','ValueType', 'UNSIGNED','Class', 'uint8','Signed', [ 0;],'Factor', [ 1;],'Offset', [ 0;],'Min', [ 0;],'Max', [ 0;],'Units', '','Comment', '','StartBit', [ 16;]),struct('Name', 'EPT_SWCU_PWR_STANDBY','Startbit', [ 0;],'SignalSize', [ 1;],'ByteOrder', 'LittleEndian','ValueType', 'UNSIGNED','Class', 'uint8','Signed', [ 0;],'Factor', [ 1;],'Offset', [ 0;],'Min', [ 0;],'Max', [ 0;],'Units', '','Comment', '','StartBit', [ 8;]),struct('Name', 'EPT_SWCU_CTRL_RC','Startbit', [ 0;],'SignalSize', [ 4;],'ByteOrder', 'LittleEndian','ValueType', 'UNSIGNED','Class', 'uint8','Signed', [ 0;],'Factor', [ 1;],'Offset', [ 0;],'Min', [ 0;],'Max', [ 0;],'Units', '','Comment', '','StartBit', [ 56;]),struct('Name', 'EPT_SWCU_CTRL_HOST_ID','Startbit', [ 0;],'SignalSize', [ 4;],'ByteOrder', 'LittleEndian','ValueType', 'UNSIGNED','Class', 'uint8','Signed', [ 0;],'Factor', [ 1;],'Offset', [ 0;],'Min', [ 0;],'Max', [ 0;],'Units', '','Comment', '','StartBit', [ 60;]),struct('Name', 'EPT_SWCU_CTRL_CHKSUM','Startbit', [ 0;],'SignalSize', [ 8;],'ByteOrder', 'LittleEndian','ValueType', 'UNSIGNED','Class', 'uint8','Signed', [ 0;],'Factor', [ 1;],'Offset', [ 0;],'Min', [ 0;],'Max', [ 0;],'Units', '','Comment', '','StartBit', [ 48;])}}
      settings: SourceProductName=Raptor
  raptor_data_def1 : Raptor_lib/Data Storage/raptor_data_def  dataName='EPT_SWCU_CTRL_HOST_ID'  initValue=0  dataType=double  storage=Calibration  calVisible=on  calType=Measurement  calDispType=Number  calEnum={'False', 'True'}  calGain=1.0  calOffset=0  calMin=-inf  calMax=inf  calFormat='-1'  calUnit=''  calHelp=''  calAccess=1  calFunction=raptor_xcp_function(gcb)  calDispHeaders=off  calColHeaders={'Col1' 'Col2' 'Col3'}  calRowHeaders={'Row1' 'Row2' 'Row3'}
      settings: SourceProductName=Raptor
  raptor_data_def2 : Raptor_lib/Data Storage/raptor_data_def  dataName='EPT_SWCU_OUTPUT_MODE'  initValue=1  dataType=double  storage=Calibration  calVisible=on  calType=Measurement  calDispType=Number  calEnum={'False', 'True'}  calGain=1.0  calOffset=0  calMin=-inf  calMax=inf  calFormat='-1'  calUnit=''  calHelp=''  calAccess=1  calFunction=raptor_xcp_function(gcb)  calDispHeaders=off  calColHeaders={'Col1' 'Col2' 'Col3'}  calRowHeaders={'Row1' 'Row2' 'Row3'}
      settings: SourceProductName=Raptor
  raptor_data_def3 : Raptor_lib/Data Storage/raptor_data_def  dataName='EPT_SWCU_POUT_CMD'  initValue=0  dataType=double  storage=Calibration  calVisible=on  calType=Measurement  calDispType=Number  calEnum={'False', 'True'}  calGain=1.0  calOffset=0  calMin=-inf  calMax=inf  calFormat='-1'  calUnit=''  calHelp=''  calAccess=1  calFunction=raptor_xcp_function(gcb)  calDispHeaders=off  calColHeaders={'Col1' 'Col2' 'Col3'}  calRowHeaders={'Row1' 'Row2' 'Row3'}
      settings: SourceProductName=Raptor
  raptor_data_def4 : Raptor_lib/Data Storage/raptor_data_def  dataName='EPT_BPSWU_SWAP_LVL'  initValue=30  dataType=double  storage=Calibration  calVisible=on  calType=Measurement  calDispType=Number  calEnum={'False', 'True'}  calGain=1.0  calOffset=0  calMin=-inf  calMax=inf  calFormat='-1'  calUnit=''  calHelp=''  calAccess=1  calFunction=raptor_xcp_function(gcb)  calDispHeaders=off  calColHeaders={'Col1' 'Col2' 'Col3'}  calRowHeaders={'Row1' 'Row2' 'Row3'}
      settings: SourceProductName=Raptor
  raptor_data_def5 : Raptor_lib/Data Storage/raptor_data_def  dataName='EPT_SWCU_CTRL_CHKSUM'  initValue=0  dataType=double  storage=Calibration  calVisible=on  calType=Measurement  calDispType=Number  calEnum={'False', 'True'}  calGain=1.0  calOffset=0  calMin=-inf  calMax=inf  calFormat='-1'  calUnit=''  calHelp=''  calAccess=1  calFunction=raptor_xcp_function(gcb)  calDispHeaders=off  calColHeaders={'Col1' 'Col2' 'Col3'}  calRowHeaders={'Row1' 'Row2' 'Row3'}
      settings: SourceProductName=Raptor
  raptor_data_def6 : Raptor_lib/Data Storage/raptor_data_def  dataName='EPT_SWCU_CTRL_RC'  initValue=0  dataType=double  storage=Calibration  calVisible=on  calType=Measurement  calDispType=Number  calEnum={'False', 'True'}  calGain=1.0  calOffset=0  calMin=-inf  calMax=inf  calFormat='-1'  calUnit=''  calHelp=''  calAccess=1  calFunction=raptor_xcp_function(gcb)  calDispHeaders=off  calColHeaders={'Col1' 'Col2' 'Col3'}  calRowHeaders={'Row1' 'Row2' 'Row3'}
      settings: SourceProductName=Raptor
  raptor_data_def7 : Raptor_lib/Data Storage/raptor_data_def  dataName='EPT_SWCU_PWR_STANDBY'  initValue=1  dataType=boolean  storage=Calibration  calVisible=on  calType=Measurement  calDispType=Number  calEnum={'False', 'True'}  calGain=1.0  calOffset=0  calMin=-inf  calMax=inf  calFormat='-1'  calUnit=''  calHelp=''  calAccess=1  calFunction=raptor_xcp_function(gcb)  calDispHeaders=off  calColHeaders={'Col1' 'Col2' 'Col3'}  calRowHeaders={'Row1' 'Row2' 'Row3'}
      settings: SourceProductName=Raptor
  raptor_data_def8 : Raptor_lib/Data Storage/raptor_data_def  dataName='EPT_SWCU_HV_ENA'  initValue=0  dataType=boolean  storage=Calibration  calVisible=on  calType=Measurement  calDispType=Number  calEnum={'False', 'True'}  calGain=1.0  calOffset=0  calMin=-inf  calMax=inf  calFormat='-1'  calUnit=''  calHelp=''  calAccess=1  calFunction=raptor_xcp_function(gcb)  calDispHeaders=off  calColHeaders={'Col1' 'Col2' 'Col3'}  calRowHeaders={'Row1' 'Row2' 'Row3'}
      settings: SourceProductName=Raptor
  raptor_data_read1 : Raptor_lib/Data Storage/raptor_data_read  dataName='EPT_SWCU_CTRL_HOST_ID'  dataShape=Scalar  idxSource=Input  idxRow=1  idxCol=1
      settings: SourceProductName=Raptor
  raptor_data_read10 : Raptor_lib/Data Storage/raptor_data_read  dataName='Flag_HV_Drive_Relay_On'  dataShape=Scalar  idxSource=Input  idxRow=1  idxCol=1
      settings: SourceProductName=Raptor
  raptor_data_read11 : Raptor_lib/Data Storage/raptor_data_read  dataName='HV_Off'  dataShape=Scalar  idxSource=Input  idxRow=1  idxCol=1
      settings: SourceProductName=Raptor
  raptor_data_read12 : Raptor_lib/Data Storage/raptor_data_read  dataName='EPT_EW_STA'  dataShape=Scalar  idxSource=Input  idxRow=1  idxCol=1
      settings: SourceProductName=Raptor
  raptor_data_read13 : Raptor_lib/Data Storage/raptor_data_read  dataName='EPT_SWCU_PWR_STANDBY'  dataShape=Scalar  idxSource=Input  idxRow=1  idxCol=1
      settings: SourceProductName=Raptor
  raptor_data_read14 : Raptor_lib/Data Storage/raptor_data_read  dataName='Flag_HV_Negative_Relay_On'  dataShape=Scalar  idxSource=Input  idxRow=1  idxCol=1
      settings: SourceProductName=Raptor
  raptor_data_read15 : Raptor_lib/Data Storage/raptor_data_read  dataName='Relay_BMS_SWU'  dataShape=Scalar  idxSource=Input  idxRow=1  idxCol=1
      settings: SourceProductName=Raptor
  raptor_data_read16 : Raptor_lib/Data Storage/raptor_data_read  dataName='Flag_Drive_Mode'  dataShape=Scalar  idxSource=Input  idxRow=1  idxCol=1
      settings: SourceProductName=Raptor
  raptor_data_read2 : Raptor_lib/Data Storage/raptor_data_read  dataName='EPT_SWCU_OUTPUT_MODE'  dataShape=Scalar  idxSource=Input  idxRow=1  idxCol=1
      settings: SourceProductName=Raptor
  raptor_data_read3 : Raptor_lib/Data Storage/raptor_data_read  dataName='HV_Setup_State'  dataShape=Scalar  idxSource=Input  idxRow=1  idxCol=1
      settings: SourceProductName=Raptor
  raptor_data_read4 : Raptor_lib/Data Storage/raptor_data_read  dataName='EPT_BPSWU_SWAP_LVL'  dataShape=Scalar  idxSource=Input  idxRow=1  idxCol=1
      settings: SourceProductName=Raptor
  raptor_data_read5 : Raptor_lib/Data Storage/raptor_data_read  dataName='EPT_SWCU_CTRL_CHKSUM'  dataShape=Scalar  idxSource=Input  idxRow=1  idxCol=1
      settings: SourceProductName=Raptor
  raptor_data_read6 : Raptor_lib/Data Storage/raptor_data_read  dataName='EPT_SWCU_CTRL_RC'  dataShape=Scalar  idxSource=Input  idxRow=1  idxCol=1
      settings: SourceProductName=Raptor
  raptor_data_read7 : Raptor_lib/Data Storage/raptor_data_read  dataName='EPT_EW_STA'  dataShape=Scalar  idxSource=Input  idxRow=1  idxCol=1
      settings: SourceProductName=Raptor
  raptor_data_read8 : Raptor_lib/Data Storage/raptor_data_read  dataName='EPT_READY'  dataShape=Scalar  idxSource=Input  idxRow=1  idxCol=1
      settings: SourceProductName=Raptor
  raptor_data_read9 : Raptor_lib/Data Storage/raptor_data_read  dataName='EPT_SWCU_HV_ENA'  dataShape=Scalar  idxSource=Input  idxRow=1  idxCol=1
      settings: SourceProductName=Raptor
  raptor_data_write16 : Raptor_lib/Data Storage/raptor_data_write  dataName='EPT_SWCU_HV_ENA'  dataShape=Scalar  idxSource=Input Port  idxRow=1  idxCol=1
      settings: SourceProductName=Raptor
  raptor_data_write20 : Raptor_lib/Data Storage/raptor_data_write  dataName='EPT_SWCU_CTRL_RC'  dataShape=Scalar  idxSource=Input Port  idxRow=1  idxCol=1
      settings: SourceProductName=Raptor
  raptor_override : Raptor_lib/Data Storage/raptor_override  paramName='Cal_EPT_SWCU_POUT_CMD'  nameSource=Parameter  measurement=None  calDispType=Number  calEnum={'False', 'True'}  calGain=1.0  calOffset=0.0  calMax=inf  calMin=-inf  calFormat='-1'  calUnit=''  calHelp=''  calAccess=1  calFunction=[raptor_xcp_function(gcb) '|' raptor_get_param_eval(gcb, 'paramName') '_Override']
      settings: SourceProductName=Raptor
  raptor_override1 : Raptor_lib/Data Storage/raptor_override  paramName='Cal_EPT_SWCU_HV_ENA'  nameSource=Parameter  measurement=None  calDispType=Number  calEnum={'False', 'True'}  calGain=1.0  calOffset=0.0  calMax=inf  calMin=-inf  calFormat='-1'  calUnit=''  calHelp=''  calAccess=1  calFunction=[raptor_xcp_function(gcb) '|' raptor_get_param_eval(gcb, 'paramName') '_Override']
      settings: SourceProductName=Raptor
  wires:
  raptor_data_read1/1 -> raptor_can_txmsg/11
  raptor_data_read6/1 -> raptor_can_txmsg/10
  EPT_SWCU_POUT_CMD/1(EPT_SWCU_POUT_CMD) -> raptor_override/1
  raptor_data_read5/1 -> raptor_can_txmsg/9
  raptor_data_read2/1 -> raptor_can_txmsg/6
  raptor_data_read4/1 -> raptor_can_txmsg/8
  raptor_data_read8/1 -> raptor_can_txmsg/1
  raptor_data_read7/1 -> raptor_can_txmsg/2
  raptor_data_read12/1 -> Logical Operator2/1
  raptor_data_read14/1 -> Logical Operator3/1
  raptor_data_read11/1 -> Logical Operator2/2
  Logical Operator3/1 -> Logical Operator4/2
  raptor_data_read10/1 -> Logical Operator3/2
  Logical Operator2/1 -> Logical Operator4/1
  raptor_data_read9/1 -> raptor_override1/1
  raptor_data_read13/1 -> raptor_can_txmsg/3
  Logical Operator4/1 -> raptor_can_txmsg/5
  Constant7/1 -> RollingCount1/1(In1)
  RollingCount1/1(Out1) -> raptor_data_write20/1
  raptor_override/1 -> raptor_can_txmsg/7
  raptor_override1/1 -> raptor_can_txmsg/4
  raptor_data_read15/1 -> Compare To Constant1/1
  Delay/1(Output) -> Latch/1(Latch)
  raptor_adjustment/1 -> Delay/2(TimeCount)
  NOT/1 -> Latch/2(Reset)
  Latch/1(Output) -> raptor_data_write16/1
  raptor_data_read3/1 -> Compare To Constant/1
  Compare To Constant/1 -> Logical Operator/1
  Logical Operator/1 -> NOT/1, Delay/1(Condition)
  Compare To Constant1/1 -> Logical Operator/2
  raptor_data_read16/1 -> Logical Operator/3
